simulink model "dac_test"  (R2023a)
settings: Solver=FixedStepDiscrete  StartTime=0.0  StopTime=10.0  MaxStep=0.2  RelTol=1e-3
settings Model: Creator=motya  LastModifiedBy=motya

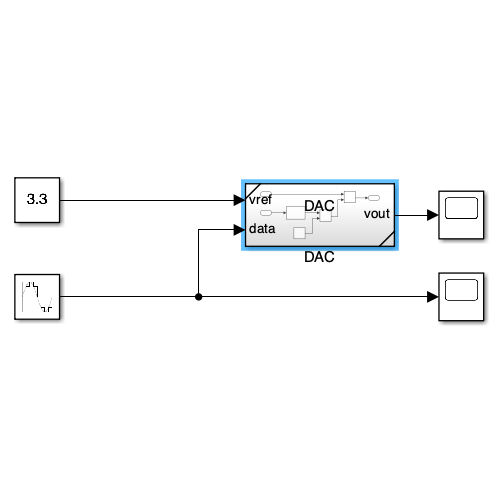
[thumbnail: Simulink's stored preview of the top-level diagram]
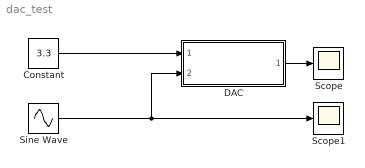
== system dac_test ==
  Constant : Constant  Value=3.3
  DAC : Subsystem  ReferencedSubsystem=DAC
  Scope : Scope
  Scope1 : Scope
  Sine Wave : Sin  Amplitude=2^3  Bias=2^3  SampleTime=0.1
  wires:
  DAC/1 -> Scope/1
  Constant/1 -> DAC/1
  Sine Wave/1 -> DAC/2, Scope1/1
